simulink model "NewModel_v3"  (R2020a)
settings: Solver=VariableStepAuto  StartTime=0.0  StopTime=1000  FixedStep=0.1  RelTol=1e-3
values from neighbouring files (symbols this model uses):
  Ctr = 1.6    [ACC_DATA.m]
  desired_distance = 10    [ACC_DATA.m]
  F_aero = 1/(2*m_Follower)*Ro_A_Cd    (= 0.00026)    [ACC_DATA.m]
  F_grav = g*sin(theta)    [ACC_DATA.m]
  F_res = g*Cr*cos(theta)    [ACC_DATA.m]
  g = 9.81    [ACC_DATA.m]
  Kb = 0.08    [ACC_DATA.m]
  Kc = 1    [ACC_DATA.m]
  m_Follower = 1500    [ACC_DATA.m]
  max_ac = 3    [ACC_DATA.m]
  min_ac = -3    [ACC_DATA.m]
  r = 0.326    [ACC_DATA.m]
  Rf = 3.28    [ACC_DATA.m]
  Rtr = 1    [ACC_DATA.m]
  time_gap = 1.4    [ACC_DATA.m]
  Tmax = 528.7 + 0.152*Ne - 0.0000217*Ne^2    (= 789.5)    [ACC_DATA.m]
  Ts = 0.1    [ACC_DATA.m]
  v0_lead = 20    [ACC_DATA.m]
  verr_gain = 0.4    [ACC_DATA.m]
  vx_gain = 0.1    [ACC_DATA.m]
  x0_ego = 10    [ACC_DATA.m]
  x0_lead = 500    [ACC_DATA.m]
  xerr_gain = 0.8    [ACC_DATA.m]
undefined symbols (not defined in the file or in its folder): ACC_model, sigbuilder_block
libraries: simulink x3, autolibshared x1
settings Model: SimulationMode=accelerator  Creator=91968  LastModifiedBy=91968

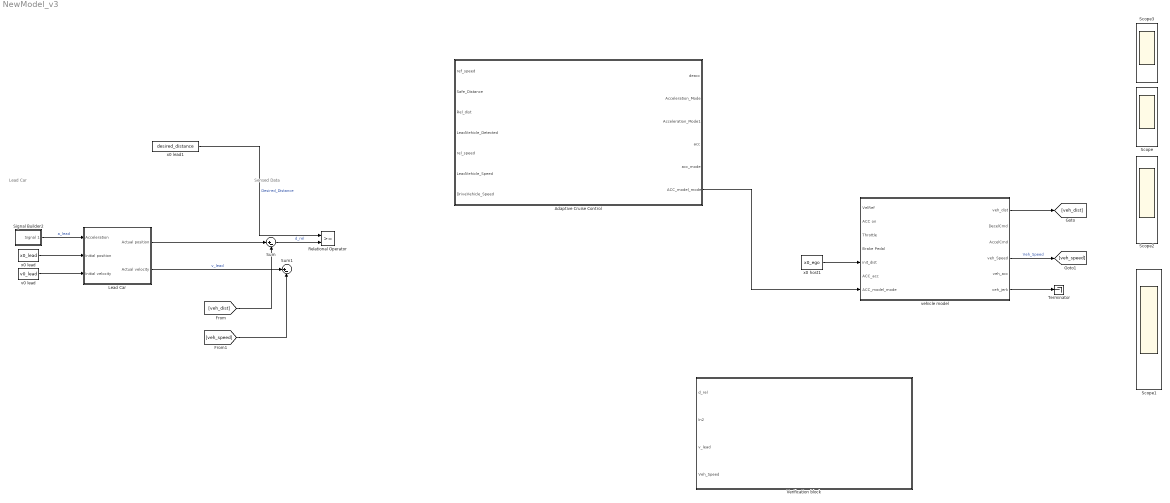
== system NewModel_v3 ==
  note: Lead Car
  note: Sensed Data
  Adaptive Cruise Control : Subsystem
      mask Display: image('index.jpg'); % Use "Edit Image" on toolstrip to change.
  Lead Car : Subsystem
  Relational Operator : RelationalOperator  OutDataTypeStr=boolean  RndMeth=Simplest
  Scope{,1..3} (4 alike) : Scope  NumInputPorts=4
  Signal Builder2 : Subsystem  Tag=STV Subsys  LoadFcn=sigbuilder_block('load');  StartFcn=sigbuilder_block('start');  StopFcn=sigbuilder_block('stop');  ClipboardFcn=sigbuilder_block('clipboard');  mask(Sigbuilder block){tuvar=[0:10]}
      mask help: Simulink:masks:SigbuilderBlock_MD
      mask init:
      | if ~strcmp(get_param(bdroot(gcbh),'SimulationStatus'),'stopped') tuvar = sigbuilder_block('maskInit'); end
      settings: CopyFcn=sigbuilder_block('copy');  DeleteFcn=sigbuilder_block('delete');  ModelCloseFcn=sigbuilder_block('modelClose');  PreSaveFcn=sigbuilder_block('preSave');  PauseFcn=sigbuilder_block('pause');  ContinueFcn=sigbuilder_block('continue');  NameChangeFcn=sigbuilder_block('namechange');  OpenFcn=sigbuilder_block('open',[-1359 225 891.75 468.75 ]);  CloseFcn=sigbuilder_block('close');
      mask Display: plot(0, 0, 100, 100,[2, 2, 32, 32, 2], [68, 8, 8, 68, 68],[32, 2], [38, 38], [32, 19, 2],[53, 60, 44], [32, 17, 17, 2],[16, 16, 31, 31]);txt = getActiveGroup(gcbh);text(2, 100, txt,'verticalAlignment', 'top');
  Sum : Sum  Inputs=|+-
  Sum1 : Sum  Inputs=|+-
  Terminator : Terminator
  Verification block : Subsystem
  v0 lead : Constant  Value=v0_lead  SampleTime=Ts
  vehicle model : Subsystem
      mask Display: image('Volvo-S60-130220211541.jpg'); % Use "Edit Image" on toolstrip to change.
  x0 host1 : Constant  Value=x0_ego  SampleTime=Ts
  x0 lead : Constant  Value=x0_lead  SampleTime=Ts
  x0 lead1 : Constant  Value=desired_distance  SampleTime=Ts
  wires:
  x0 lead/1 -> Lead Car/2(Initial position)
  v0 lead/1 -> Lead Car/3(Initial velocity)
  Signal Builder2/1(Signal 1) -> Lead Car/1(Acceleration)  "a_lead"
  Lead Car/1(Actual position) -> Sum/1
  Lead Car/2(Actual velocity) -> Sum1/1  "v_lead"
  x0 lead1/1 -> Relational Operator/1  "Desired_Distance"
  Sum/1 -> Relational Operator/2  "d_rel"
  ? -> Verification block/2(In2)
  ? -> vehicle model/1(VelRef)  "<>"
  ? -> vehicle model/2(ACC on)
  ? -> vehicle model/3(Throttle)
  ? -> vehicle model/4(Brake Pedal)
  x0 host1/1 -> vehicle model/5(init_dist)
  vehicle model/6(veh_jerk) -> Terminator/1
  vehicle model/1(veh_dist) -> [veh_dist]
  [veh_dist] -> Sum/2
  [veh_speed] -> Sum1/2
  vehicle model/4(veh_Speed) -> [veh_speed]  "Veh_Speed"
  Adaptive Cruise Control/6(ACC_model_mode) -> vehicle model/7(ACC_model_mode)

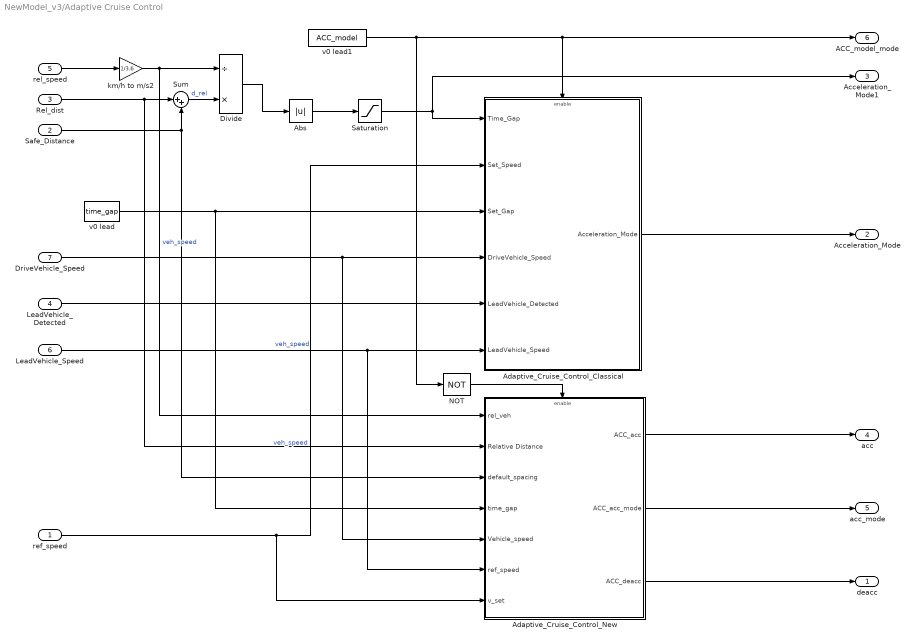
== system NewModel_v3/Adaptive Cruise Control ==
  ref_speed : Inport
  Safe_Distance : Inport  Port=2
  Rel_dist : Inport  Port=3
  LeadVehicle_Detected : Inport  Port=4  OutMin=0  OutMax=1
  rel_speed : Inport  Port=5  OutMin=0  OutMax=1
  LeadVehicle_Speed : Inport  Port=6  OutMin=0  OutMax=255
  DriveVehicle_Speed : Inport  Port=7  OutMin=0  OutMax=255
  Abs : Abs
  Adaptive_Cruise_Control_Classical : Subsystem
  Adaptive_Cruise_Control_New : Subsystem
  Divide : Product  Inputs=/*
  NOT : Logic  Operator=NOT  IconShape=distinctive  AllPortsSameDT=off  OutDataTypeStr=boolean
  Saturation : Saturate  UpperLimit=100  LowerLimit=0
  Sum : Sum  Inputs=|++
  km/h to m/s2 : Gain  Gain=1/3.6
  v0 lead : Constant  Value=time_gap  SampleTime=Ts
  v0 lead1 : Constant  Value=ACC_model  SampleTime=Ts
  deacc : Outport
  Acceleration_Mode : Outport  Port=2
  Acceleration_Mode1 : Outport  Port=3
  acc : Outport  Port=4
  acc_mode : Outport  Port=5
  ACC_model_mode : Outport  Port=6
  wires:
  Adaptive_Cruise_Control_Classical/1(Acceleration_Mode) -> Acceleration_Mode/1
  DriveVehicle_Speed/1 -> Adaptive_Cruise_Control_New/5(Vehicle_speed), Adaptive_Cruise_Control_Classical/4(DriveVehicle_Speed)
  Saturation/1 -> Acceleration_Mode1/1, Adaptive_Cruise_Control_Classical/1(Time_Gap)
  v0 lead/1 -> Adaptive_Cruise_Control_New/4(time_gap), Adaptive_Cruise_Control_Classical/3(Set_Gap)
  LeadVehicle_Detected/1 -> Adaptive_Cruise_Control_Classical/5(LeadVehicle_Detected)
  Divide/1 -> Abs/1
  Rel_dist/1 -> Adaptive_Cruise_Control_New/2(Relative Distance), Sum/1
  rel_speed/1 -> km/h to m/s2/1
  Abs/1 -> Saturation/1
  Safe_Distance/1 -> Adaptive_Cruise_Control_New/3(default_spacing), Sum/2
  Sum/1 -> Divide/2  "d_rel"
  Adaptive_Cruise_Control_New/3(ACC_deacc) -> deacc/1
  LeadVehicle_Speed/1 -> Adaptive_Cruise_Control_New/6(ref_speed), Adaptive_Cruise_Control_Classical/6(LeadVehicle_Speed)  "veh_speed"
  ref_speed/1 -> Adaptive_Cruise_Control_New/7(v_set), Adaptive_Cruise_Control_Classical/2(Set_Speed)  "veh_speed"
  km/h to m/s2/1 -> Adaptive_Cruise_Control_New/1(rel_veh), Divide/1  "veh_speed"
  Adaptive_Cruise_Control_New/1(ACC_acc) -> acc/1
  Adaptive_Cruise_Control_New/2(ACC_acc_mode) -> acc_mode/1
  v0 lead1/1 -> ACC_model_mode/1, Adaptive_Cruise_Control_Classical/Enable, NOT/1
  NOT/1 -> Adaptive_Cruise_Control_New/Enable

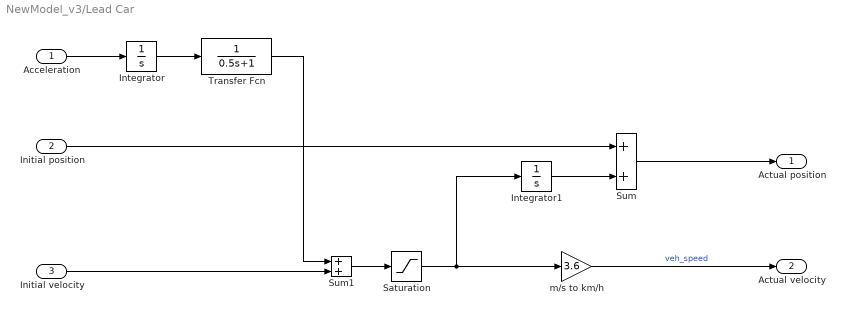
== system NewModel_v3/Lead Car ==
  Acceleration : Inport
  Initial position : Inport  Port=2
  Initial velocity : Inport  Port=3
  Integrator : Integrator
  Integrator1 : Integrator
  Saturation : Saturate  UpperLimit=200  LowerLimit=0
  Sum : Sum
  Sum1 : Sum
  Transfer Fcn : TransferFcn  Denominator=[0.5 1]
  m/s to km/h : Gain  Gain=3.6
  Actual position : Outport  VectorParamsAs1DForOutWhenUnconnected=off
  Actual velocity : Outport  Port=2  VectorParamsAs1DForOutWhenUnconnected=off
  wires:
  Transfer Fcn/1 -> Sum1/1
  Initial velocity/1 -> Sum1/2
  Integrator/1 -> Transfer Fcn/1
  Sum1/1 -> Saturation/1
  Acceleration/1 -> Integrator/1
  Initial position/1 -> Sum/1
  Integrator1/1 -> Sum/2
  Saturation/1 -> Integrator1/1, m/s to km/h/1
  Sum/1 -> Actual position/1
  m/s to km/h/1 -> Actual velocity/1  "veh_speed"

== system NewModel_v3/Signal Builder2 ==
  Demux : Demux  Tag=STV Demux  Outputs=1
      settings: DisplayOption=none
  FromWs : FromWorkspace  Tag=STV FromWs  VariableName=tuvar
      SigBuilderData=|
      | common.afterFinalStr = 'Extrapolate'
      | common.sampleTime = 0
      | dataSet.timeRange = [0 1000]
      | dataSet.name = 'Group 1'
      | sbobj.Groups.Name = 'Group 1'
      | sbobj.Groups.Signals.Name = 'Signal 1'
      | sbobj.Groups.Signals.XData = [0 20 30 40 60 80 100 126 150 200 250 300 350 400 451 502 539 549 599 650 700 749 799 847 902 956 1000]
      | sbobj.Groups.Signals.YData = [0.07 0.14 0.25 0.21 0.385 0.248 -0.09 0.032 0.006 -0.104 -0.092 -0.202 -0.182 -0.072 0.044 0.092 0.146 0.116 0.258 0.292 0.178 0.004 -0.132 -0.224 -0.124 -0.07 0]
      | sbobj.Groups.TimeRange = [0 1000]
  Signal 1 : Outport  Tag=STV Outport
  wires:
  Demux/1 -> Signal 1/1
  FromWs/1 -> Demux/1

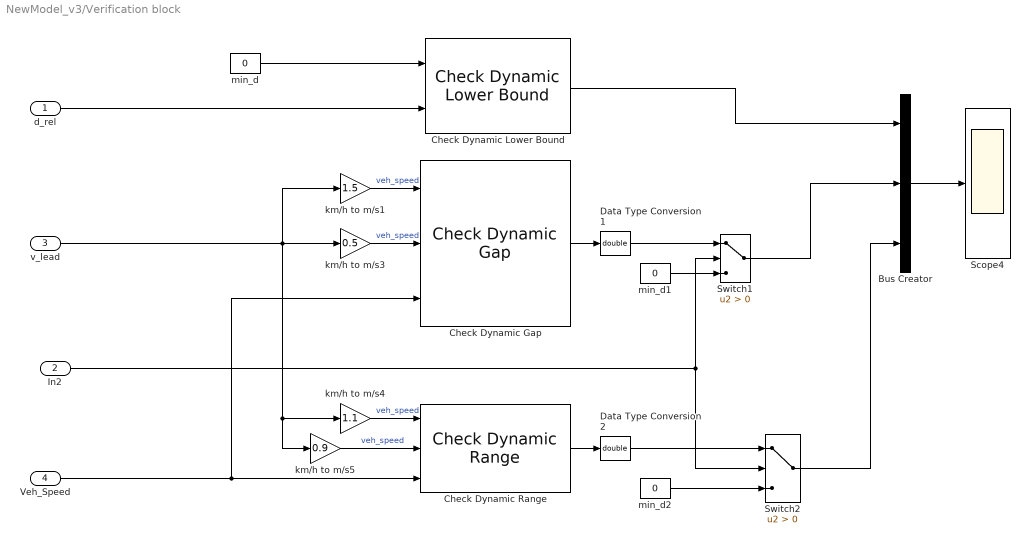
== system NewModel_v3/Verification block ==
  d_rel : Inport
  In2 : Inport  Port=2
  v_lead : Inport  Port=3
  Veh_Speed : Inport  Port=4
  Bus Creator : BusCreator  Inputs=3
  Check Dynamic Gap : simulink/Model Verification/Check  Dynamic Gap  Description=u < min || max < u  enabled=on  stopWhenAssertionFail=off  export=on  icon=graphic
      settings: SourceProductBaseCode=SL
  Check Dynamic Range : simulink/Model Verification/Check  Dynamic Range  Description=min < u < max  enabled=on  stopWhenAssertionFail=off  export=on  icon=graphic
      settings: SourceProductBaseCode=SL
  Check Dynamic Lower Bound : simulink/Model Verification/Check Dynamic  Lower Bound  Description=min < u  Enabled=on  stopWhenAssertionFail=off  export=on  icon=graphic
      settings: SourceProductBaseCode=SL
  Data Type Conversion1 : DataTypeConversion  OutDataTypeStr=double
  Data Type Conversion2 : DataTypeConversion  OutDataTypeStr=double
  Scope4 : Scope
  Switch1 : Switch  Criteria=u2 > Threshold  SaturateOnIntegerOverflow=on  InputSameDT=on
  Switch2 : Switch  Criteria=u2 > Threshold  SaturateOnIntegerOverflow=on  InputSameDT=on
  km/h to m/s1 : Gain  Gain=1.5
  km/h to m/s3 : Gain  Gain=0.5
  km/h to m/s4 : Gain  Gain=1.1
  km/h to m/s5 : Gain  Gain=0.9
  min_d : Constant  Value=0
  min_d1 : Constant  Value=0
  min_d2 : Constant  Value=0
  wires:
  min_d1/1 -> Switch1/3
  Check Dynamic Range/1 -> Data Type Conversion2/1
  min_d2/1 -> Switch2/3
  Data Type Conversion2/1 -> Switch2/1
  km/h to m/s3/1 -> Check Dynamic Gap/2  "veh_speed"
  Data Type Conversion1/1 -> Switch1/1
  Switch1/1 -> Bus Creator/2
  Switch2/1 -> Bus Creator/3
  km/h to m/s5/1 -> Check Dynamic Range/2  "veh_speed"
  min_d/1 -> Check Dynamic Lower Bound/1
  km/h to m/s4/1 -> Check Dynamic Range/1  "veh_speed"
  v_lead/1 -> km/h to m/s4/1, km/h to m/s5/1, km/h to m/s3/1, km/h to m/s1/1
  In2/1 -> Switch2/2, Switch1/2
  Check Dynamic Gap/1 -> Data Type Conversion1/1
  Check Dynamic Lower Bound/1 -> Bus Creator/1
  km/h to m/s1/1 -> Check Dynamic Gap/1  "veh_speed"
  Veh_Speed/1 -> Check Dynamic Gap/3, Check Dynamic Range/3
  d_rel/1 -> Check Dynamic Lower Bound/2
  Bus Creator/1 -> Scope4/1

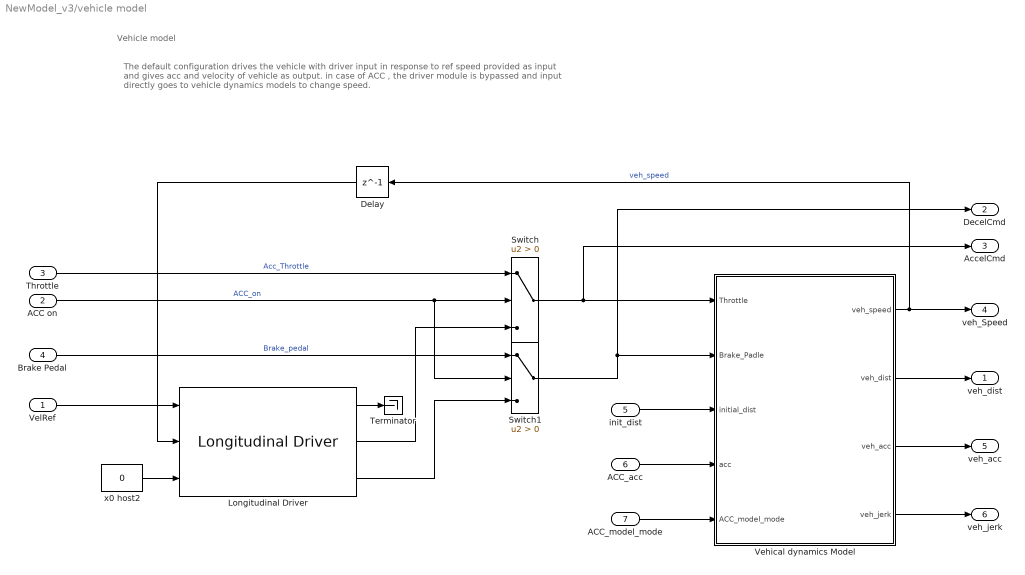
== system NewModel_v3/vehicle model ==
  note: Vehicle model
  note: The default configuration drives the vehicle with driver input in response to ref speed provided as input and gives acc and velocity of vehicle as output.
      | in case of ACC , the driver module is bypassed and input directly goes to vehicle dynamics models to change speed.
  VelRef : Inport
  ACC on : Inport  Port=2
  Throttle : Inport  Port=3
  Brake Pedal : Inport  Port=4
  init_dist : Inport  Port=5
  ACC_acc : Inport  Port=6
  ACC_model_mode : Inport  Port=7
  Delay : Delay  DelayLength=1  InitialCondition=0
  Longitudinal Driver : autolibshared/Longitudinal Driver  extAccelOvr=off  extDecelOvr=off  extAccelHld=off  extDecelHld=off  extAccelZero=off  extDecelZero=off  cntrlType=PI  shftType=None  velUnits=m/s  gearOut=off  Kp=15  Ki=1  Kff=.05  Kg=.01  VehVelVec=[0 100]  KffVec=[.1 .1]  KpVec=[10 10]  KiVec=[5 5]  KgVec=[0 0]  m=1500  Kpt=3000  tau=.1  L=2  aR=200  bR=2.5  cR=.5  g=9.81  vnom=100  Kaw=.1  tauerr=.03  tauPt=2  GearInit=0  tShift=.1  pdlVec=[0.1 0.4 0.5 0.9]  upShftTbl=[-1 12.9375 26.4375 39.9375 51.18749999999999 62.4375 72.84375 83.25;-1 16.3125 29.8125 43.3125 54.5624 65.8125 76.78125 87.75;-1 19.6875 33.1875 46.68749999999999 57.9375 69.1875 80.71875 92.25;-1 33 52.5 77.25 100.5 138.75 161.875 185]  dwnShftTbl=[1 9.5625 23.0625 36.5625 47.8125 59.0625 68.90625 78.75;1 12.9375 26.4375 39.9375 51.18749999999999 62.4375 72.84375 83.25;1 16.3125 29.8125 43.3125 54.562499 65.8125 76.78125 87.75;1 19.6875 33.1875 46.68749999999999 57.9375 69.1875 80.71875 92.25]  tClutch=.5  tRev=.5  tPark=120  aMode=1  UpGearVec="[0  1  2  3  4  5  6  7]"  DownGearVec="[1  2  3  4  5  6  7  8]"
      settings: SourceProductBaseCode=PW,MT,VE,VP
  Switch : Switch  Criteria=u2 > Threshold  SaturateOnIntegerOverflow=on  InputSameDT=on
  Switch1 : Switch  Criteria=u2 > Threshold  SaturateOnIntegerOverflow=on  InputSameDT=on
  Terminator : Terminator
  Vehical dynamics Model : Subsystem
  x0 host2 : Constant  Value=0  SampleTime=Ts
  veh_dist : Outport
  DecelCmd : Outport  Port=2
  AccelCmd : Outport  Port=3
  veh_Speed : Outport  Port=4
  veh_acc : Outport  Port=5
  veh_jerk : Outport  Port=6
  wires:
  VelRef/1 -> Longitudinal Driver/1
  Vehical dynamics Model/2(veh_dist) -> veh_dist/1
  init_dist/1 -> Vehical dynamics Model/3(initial_dist)
  Delay/1 -> Longitudinal Driver/2
  x0 host2/1 -> Longitudinal Driver/3
  Vehical dynamics Model/1(veh_speed) -> Delay/1, veh_Speed/1  "veh_speed"
  Vehical dynamics Model/4(veh_jerk) -> veh_jerk/1
  Vehical dynamics Model/3(veh_acc) -> veh_acc/1
  Longitudinal Driver/1 -> Terminator/1
  ACC on/1 -> Switch1/2, Switch/2  "ACC_on"
  Longitudinal Driver/2 -> Switch/3
  Switch1/1 -> DecelCmd/1, Vehical dynamics Model/2(Brake_Padle)
  Switch/1 -> AccelCmd/1, Vehical dynamics Model/1(Throttle)
  Longitudinal Driver/3 -> Switch1/3
  Throttle/1 -> Switch/1  "Acc_Throttle"
  Brake Pedal/1 -> Switch1/1  "Brake_pedal"
  ACC_acc/1 -> Vehical dynamics Model/4(acc)
  ACC_model_mode/1 -> Vehical dynamics Model/5(ACC_model_mode)

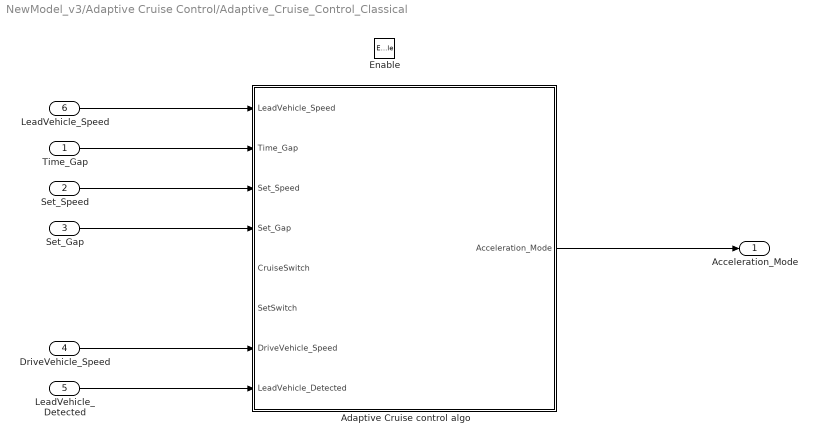
== system NewModel_v3/Adaptive Cruise Control/Adaptive_Cruise_Control_Classical ==
  Time_Gap : Inport
  Set_Speed : Inport  Port=2
  Set_Gap : Inport  Port=3
  DriveVehicle_Speed : Inport  Port=4  OutMin=0  OutMax=255
  LeadVehicle_Detected : Inport  Port=5  OutMin=0  OutMax=1
  LeadVehicle_Speed : Inport  Port=6  OutMin=0  OutMax=255
  Enable : EnablePort
  Adaptive Cruise control algo : Stateflow chart  RequirementInfo={} %GIDa_57645b32_15f0_49df_b2ac_141007f7ec66  TreatAsAtomicUnit=on
  Acceleration_Mode : Outport  OutMin=0  OutMax=255
  wires:
  LeadVehicle_Speed/1 -> Adaptive Cruise control algo/1(LeadVehicle_Speed)
  Set_Gap/1 -> Adaptive Cruise control algo/4(Set_Gap)
  Set_Speed/1 -> Adaptive Cruise control algo/3(Set_Speed)
  Time_Gap/1 -> Adaptive Cruise control algo/2(Time_Gap)
  LeadVehicle_Detected/1 -> Adaptive Cruise control algo/8(LeadVehicle_Detected)
  DriveVehicle_Speed/1 -> Adaptive Cruise control algo/7(DriveVehicle_Speed)
  Adaptive Cruise control algo/1(Acceleration_Mode) -> Acceleration_Mode/1

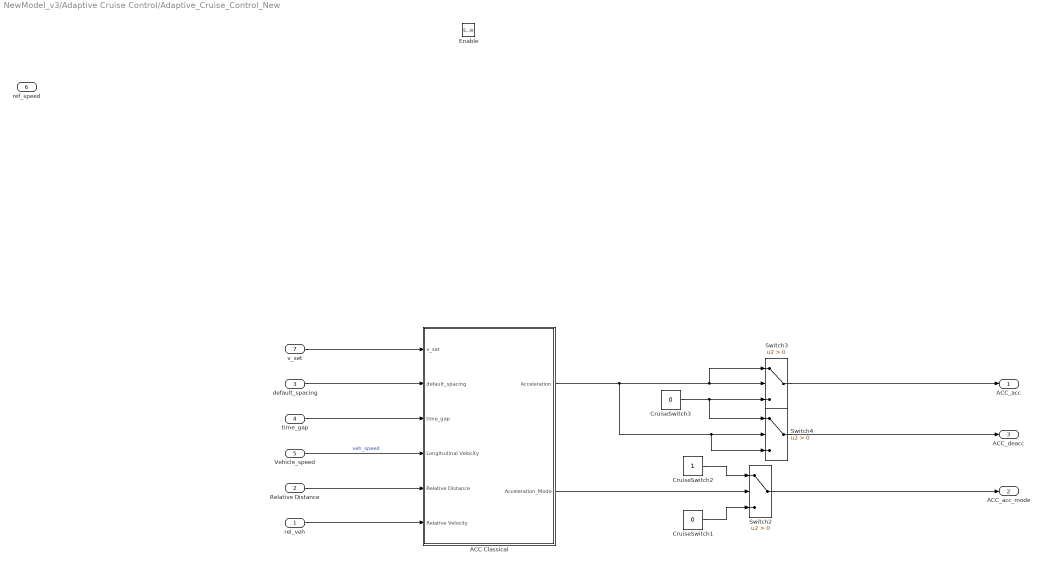
== system NewModel_v3/Adaptive Cruise Control/Adaptive_Cruise_Control_New ==
  rel_veh : Inport
  Relative Distance : Inport  Port=2
  default_spacing : Inport  Port=3
  time_gap : Inport  Port=4
  Vehicle_speed : Inport  Port=5
  ref_speed : Inport  Port=6
  v_set : Inport  Port=7
  Enable : EnablePort
  ACC Classical : Subsystem  TreatAsAtomicUnit=on  VariantControl=controller_type == 1
      settings: RTWFileNameOpts=Use function name
  CruiseSwitch1 : Constant  Value=0
  CruiseSwitch2 : Constant
  CruiseSwitch3 : Constant  Value=0
  Switch2 : Switch  Criteria=u2 > Threshold
  Switch3 : Switch  Criteria=u2 > Threshold
  Switch4 : Switch  Criteria=u2 > Threshold
  ACC_acc : Outport
  ACC_acc_mode : Outport  Port=2
  ACC_deacc : Outport  Port=3
  wires:
  v_set/1 -> ACC Classical/1(v_set)
  Relative Distance/1 -> ACC Classical/5(Relative Distance)
  default_spacing/1 -> ACC Classical/2(default_spacing)
  time_gap/1 -> ACC Classical/3(time_gap)
  Vehicle_speed/1 -> ACC Classical/4(Longitudinal Velocity)  "veh_speed"
  rel_veh/1 -> ACC Classical/6(Relative Velocity)
  ACC Classical/2(Acceleration_Mode) -> Switch2/2
  CruiseSwitch1/1 -> Switch2/3
  CruiseSwitch2/1 -> Switch2/1
  Switch2/1 -> ACC_acc_mode/1
  ACC Classical/1(Acceleration) -> Switch4/3, Switch4/2, Switch3/1, Switch3/2
  Switch3/1 -> ACC_acc/1
  CruiseSwitch3/1 -> Switch4/1, Switch3/3
  Switch4/1 -> ACC_deacc/1

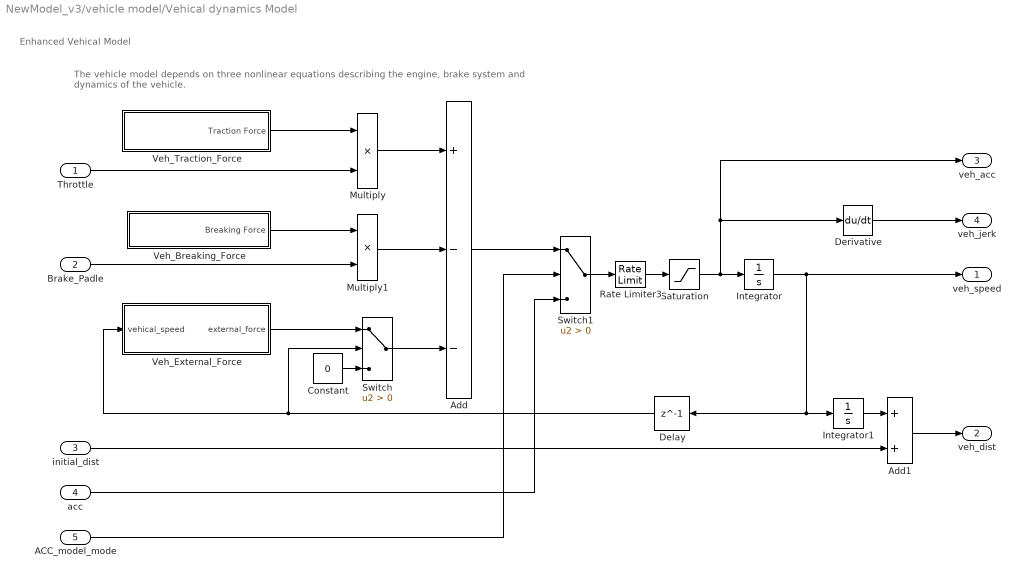
== system NewModel_v3/vehicle model/Vehical dynamics Model ==
  note: The vehicle model depends on three nonlinear equations describing the engine, brake system and dynamics of the vehicle.
  note: Enhanced Vehical Model
  Throttle : Inport
  Brake_Padle : Inport  Port=2
  initial_dist : Inport  Port=3
  acc : Inport  Port=4
  ACC_model_mode : Inport  Port=5
  Add : Sum  Inputs=+--
  Add1 : Sum
  Constant : Constant  Value=0
  Delay : Delay  DelayLength=1  InitialCondition=0
  Derivative : Derivative
  Integrator : Integrator
  Integrator1 : Integrator
  Multiply : Product
  Multiply1 : Product
  Rate Limiter3 : RateLimiter
  Saturation : Saturate  UpperLimit=3  LowerLimit=-3
  Switch : Switch  Criteria=u2 > Threshold  SaturateOnIntegerOverflow=on  InputSameDT=on
  Switch1 : Switch  Criteria=u2 > Threshold  SaturateOnIntegerOverflow=on  InputSameDT=on
  Veh_Breaking_Force : Subsystem
  Veh_External_Force : Subsystem
  Veh_Traction_Force : Subsystem
  veh_speed : Outport  VectorParamsAs1DForOutWhenUnconnected=off
  veh_dist : Outport  Port=2  VectorParamsAs1DForOutWhenUnconnected=off
  veh_acc : Outport  Port=3  VectorParamsAs1DForOutWhenUnconnected=off
  veh_jerk : Outport  Port=4  VectorParamsAs1DForOutWhenUnconnected=off
  wires:
  Switch/1 -> Add/3
  Brake_Padle/1 -> Multiply1/2
  Veh_Breaking_Force/1("Breaking Force ") -> Multiply1/1
  Throttle/1 -> Multiply/2
  Multiply1/1 -> Add/2
  Multiply/1 -> Add/1
  Veh_Traction_Force/1(Traction Force) -> Multiply/1
  Integrator1/1 -> Add1/1
  Add1/1 -> veh_dist/1
  initial_dist/1 -> Add1/2
  Delay/1 -> Switch/2, Veh_External_Force/1(vehical_speed)
  Veh_External_Force/1(external_force) -> Switch/1
  Constant/1 -> Switch/3
  Add/1 -> Switch1/1
  Derivative/1 -> veh_jerk/1
  Rate Limiter3/1 -> Saturation/1
  Saturation/1 -> Integrator/1, Derivative/1, veh_acc/1
  Integrator/1 -> veh_speed/1, Delay/1, Integrator1/1
  Switch1/1 -> Rate Limiter3/1
  acc/1 -> Switch1/3
  ACC_model_mode/1 -> Switch1/2

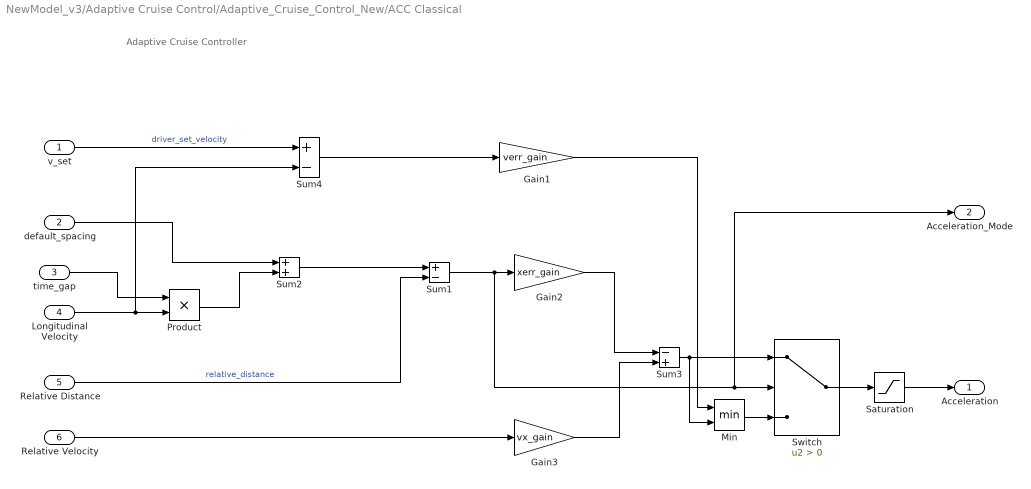
== system NewModel_v3/Adaptive Cruise Control/Adaptive_Cruise_Control_New/ACC Classical ==
  note: Adaptive Cruise Controller
  v_set : Inport
  default_spacing : Inport  Port=2
  time_gap : Inport  Port=3
  Longitudinal Velocity : Inport  Port=4
  Relative Distance : Inport  Port=5
  Relative Velocity : Inport  Port=6
  Gain1 : Gain  Gain=verr_gain
  Gain2 : Gain  Gain=xerr_gain
  Gain3 : Gain  Gain=vx_gain
  Min : MinMax  Inputs=2
  Product : Product
  Saturation : Saturate  UpperLimit=max_ac  LowerLimit=min_ac
  Sum1 : Sum  Inputs=+-
  Sum2 : Sum
  Sum3 : Sum  Inputs=-+
  Sum4 : Sum  Inputs=+-
  Switch : Switch  Criteria=u2 > Threshold
  Acceleration : Outport  VectorParamsAs1DForOutWhenUnconnected=off
  Acceleration_Mode : Outport  Port=2  VectorParamsAs1DForOutWhenUnconnected=off
  wires:
  Longitudinal Velocity/1 -> Product/2, Sum4/2
  default_spacing/1 -> Sum2/1
  Gain2/1 -> Sum3/1
  Sum4/1 -> Gain1/1
  Min/1 -> Switch/3
  Gain3/1 -> Sum3/2
  Switch/1 -> Saturation/1
  Relative Velocity/1 -> Gain3/1
  time_gap/1 -> Product/1
  Saturation/1 -> Acceleration/1
  Product/1 -> Sum2/2
  v_set/1 -> Sum4/1  "driver_set_velocity"
  Sum3/1 -> Min/2, Switch/1
  Sum1/1 -> Acceleration_Mode/1, Switch/2, Gain2/1
  Gain1/1 -> Min/1
  Relative Distance/1 -> Sum1/2  "relative_distance"
  Sum2/1 -> Sum1/1

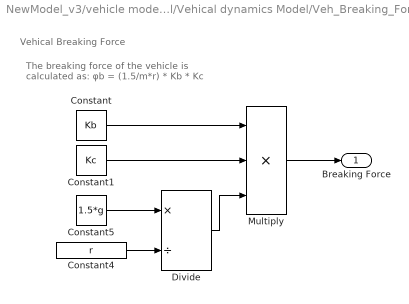
== system NewModel_v3/vehicle model/Vehical dynamics Model/Veh_Breaking_Force ==
  note: Vehical Breaking Force
  note: The breaking force of the vehicle is calculated as:
      | φb = (1.5/m*r) * Kb * Kc
  Constant : Constant  Value=Kb
  Constant1 : Constant  Value=Kc
  Constant4 : Constant  Value=r
  Constant5 : Constant  Value=1.5*g
  Divide : Product  Inputs=*/
  Multiply : Product  Inputs=3
  "Breaking Force " : Outport  VectorParamsAs1DForOutWhenUnconnected=off
  wires:
  Multiply/1 -> "Breaking Force "/1
  Constant4/1 -> Divide/2
  Constant1/1 -> Multiply/2
  Constant/1 -> Multiply/1
  Constant5/1 -> Divide/1
  Divide/1 -> Multiply/3

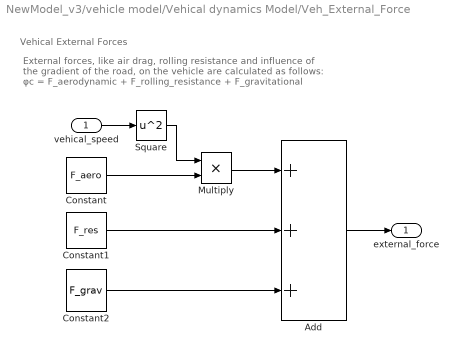
== system NewModel_v3/vehicle model/Vehical dynamics Model/Veh_External_Force ==
  note: External forces, like air drag, rolling resistance and
      | influence of the gradient of the road, on the vehicle are calculated as follows:
      |
      | φc = F_aerodynamic + F_rolling_resistance + F_gravitational
  note: Vehical External Forces
  vehical_speed : Inport
  Add : Sum  Inputs=+++
  Constant : Constant  Value=F_aero
  Constant1 : Constant  Value=F_res
  Constant2 : Constant  Value=F_grav
  Multiply : Product
  Square : Math  Operator=square  SignedPower=on  SaturateOnIntegerOverflow=on
  external_force : Outport  VectorParamsAs1DForOutWhenUnconnected=off
  wires:
  Add/1 -> external_force/1
  Constant1/1 -> Add/2
  Constant2/1 -> Add/3
  Constant/1 -> Multiply/2
  vehical_speed/1 -> Square/1
  Square/1 -> Multiply/1
  Multiply/1 -> Add/1

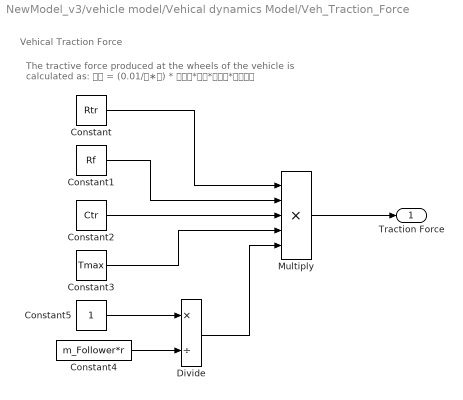
== system NewModel_v3/vehicle model/Vehical dynamics Model/Veh_Traction_Force ==
  note: The tractive force produced at the wheels of the vehicle is calculated as:
      | 𝜑𝑡 = (0.01/𝑚∗𝑟) * 𝑅𝑡𝑟*𝑅𝑓*𝐶𝑡𝑟*𝑇𝑚𝑎𝑥
  note: Vehical Traction Force
  Constant : Constant  Value=Rtr
  Constant1 : Constant  Value=Rf
  Constant2 : Constant  Value=Ctr
  Constant3 : Constant  Value=Tmax
  Constant4 : Constant  Value=m_Follower*r
  Constant5 : Constant
  Divide : Product  Inputs=*/
  Multiply : Product  Inputs=5
  Traction Force : Outport  VectorParamsAs1DForOutWhenUnconnected=off
  wires:
  Constant/1 -> Multiply/1
  Constant4/1 -> Divide/2
  Constant1/1 -> Multiply/2
  Constant5/1 -> Divide/1
  Constant3/1 -> Multiply/4
  Divide/1 -> Multiply/5
  Constant2/1 -> Multiply/3
  Multiply/1 -> Traction Force/1

== stateflow chart NewModel_v3/Adaptive Cruise Control/Adaptive_Cruise_Control_Classical/Adaptive Cruise control algo ==
  state ACC_STANDBY_MODE
    entry:
    Acceleration_Mode = 1;
  state ACC_OFF_MODE
    entry:
    Acceleration_Mode = 0;
  state ACC_ON_MODE
    state LeadVehicle_Not_Detected_Resume
      entry:
      Acceleration_Mode= 1;
    state LeadVehicle_Detected_Resume
      entry:
      Acceleration_Mode= 3;
    state LeadVehicle_Detected_Follow
      entry:
      Acceleration_Mode= 2;
    state LeadVehicle_Not_Detected
      entry:
      Acceleration_Mode= 1;
    state LeadVehicle_Speed_equal_Set_Speed
      entry:
      Acceleration_Mode= 4;
    state LeadVehicle_Speed_lessthan_Set_Speed
      entry:
      Acceleration_Mode= 5;
    (default) -> LeadVehicle_Detected_Follow
    LeadVehicle_Detected_Resume -> LeadVehicle_Not_Detected_Resume [order 1] : [LeadVehicle_Detected ==0]
    LeadVehicle_Detected_Follow -> LeadVehicle_Detected_Resume [order 3] : [(DriveVehicle_Speed==Set_Speed) ...
        | && (LeadVehicle_Speed >= Set_Speed)...
        |  && (Time_Gap>=Set_Gap)]
    LeadVehicle_Speed_lessthan_Set_Speed -> LeadVehicle_Not_Detected_Resume [order 2] : [(LeadVehicle_Detected==0) ...
        | || (DriveVehicle_Speed <= Set_Speed)]
    LeadVehicle_Detected_Resume -> LeadVehicle_Speed_lessthan_Set_Speed [order 2] : [(DriveVehicle_Speed< Set_Speed) ...
        | && (LeadVehicle_Speed > DriveVehicle_Speed)...
        | || (Time_Gap >= Set_Gap)]
    LeadVehicle_Speed_lessthan_Set_Speed -> LeadVehicle_Detected_Resume [order 1] : [(DriveVehicle_Speed< Set_Speed) ...
        | && (LeadVehicle_Speed > DriveVehicle_Speed)...
        | && (Time_Gap >= Set_Gap)]
    LeadVehicle_Detected_Follow -> LeadVehicle_Not_Detected [order 2] : [LeadVehicle_Detected ==0]
    LeadVehicle_Not_Detected -> LeadVehicle_Detected_Follow [order 1] : [(LeadVehicle_Detected==1) && ...
        | (DriveVehicle_Speed == Set_Speed) && ...
        |  (LeadVehicle_Speed >= Set_Speed) &&...
        |  (Time_Gap>=Set_Gap)]
    LeadVehicle_Detected_Follow -> LeadVehicle_Speed_equal_Set_Speed [order 1] : [(LeadVehicle_Detected==1) && ((LeadVehicle_Speed < Set_Speed) || (Time_Gap<Set_Gap))]
    LeadVehicle_Speed_equal_Set_Speed -> LeadVehicle_Not_Detected [order 1] : [(LeadVehicle_Detected==0) && ...
        | (DriveVehicle_Speed == Set_Speed)]
    LeadVehicle_Not_Detected -> LeadVehicle_Speed_equal_Set_Speed [order 2] : [(LeadVehicle_Detected==1) && ...
        | (LeadVehicle_Speed < Set_Speed) || ...
        | (Time_Gap<Set_Gap)]
    LeadVehicle_Speed_lessthan_Set_Speed -> LeadVehicle_Speed_equal_Set_Speed [order 3] : [(LeadVehicle_Speed< Set_Speed) ...
        | && (LeadVehicle_Speed < DriveVehicle_Speed)...
        | || (Time_Gap == 0.75*Set_Gap)]
    LeadVehicle_Speed_equal_Set_Speed -> LeadVehicle_Speed_lessthan_Set_Speed [order 2] : [(LeadVehicle_Speed*1.25 >= DriveVehicle_Speed) ...
        | && (LeadVehicle_Speed*0.75 <= DriveVehicle_Speed)...
        | && (DriveVehicle_Speed < Set_Speed) && (Time_Gap <=1.25*Set_Gap)...
        | && (Time_Gap >= 0.75*Set_Gap)]
  note: State
      | Description
      | Condition
      | Next State
      |
      | IDLE_STATE
      | Set cc refrence speed & set_speed equal to input speed
      | default || ACC_OFF
      | SPEED_TRACKING
      |
      | SPEED_TRACKING
      | Follow the set speed chosen by the driver
      | ACC_ON event occured && obstacle_distance < set_distance
      | DISTANCE_TRACKING / IDLE_STATE
      |
      | DISTANCE_TRACKING
      | Follow the tracking speed to keep the min distance maintained
      | obstacle_distance > set_distance...
      | && after(60,sec)
      | SPEED_TRACKING
  (default) -> ACC_OFF_MODE
  ACC_OFF_MODE -> ACC_STANDBY_MODE : [CruiseSwitch == 1]
  ACC_STANDBY_MODE -> ACC_OFF_MODE [order 1] : [CruiseSwitch==0]
  ACC_ON_MODE -> ACC_STANDBY_MODE [order 1] : [SetSwitch ==0]
  ACC_STANDBY_MODE -> ACC_ON_MODE [order 2] : [SetSwitch ==1]
  ACC_ON_MODE -> ACC_OFF_MODE [order 2] : [CruiseSwitch == 0]
  data: LeadVehicle_Speed input; Time_Gap input; Set_Speed input; Set_Gap input; CruiseSwitch input [0..1]; SetSwitch input [0..1]; DriveVehicle_Speed input; LeadVehicle_Detected input; Acceleration_Mode output
